simulink model "bldc_model_2018"  (R2018a)
settings: Solver=ode3  StartTime=0.0  StopTime=1  FixedStep=1e-3  MaxStep=0.0001  RelTol=1e-3  EnableMultiTasking=on
settings Model: Creator=root  LastModifiedBy=Rusty Goh
settings SolverCC: AlgebraicLoopSolver=LineSearch
settings DataIOCC: LimitDataPoints=on  SaveFormat=Array
settings OptimizationCC: LifeSpan=inf
settings DebuggingCC: SolverPrmCheckMsg=warning  SFUnexpectedBacktrackingDiag=warning  SFNoUnconditionalDefaultTransitionDiag=warning  SFExecutionAtInitializationDiag=none
settings HardwareCC: ProdBitPerPointer=32  ProdBitPerSizeT=32  ProdBitPerPtrDiffT=32  ProdLargestAtomicFloat=None  ProdIntDivRoundTo=Undefined  ProdEndianess=Unspecified  ProdWordSize=32  ProdHWDeviceType=32-bit Generic
settings ModelReferenceCC: PropagateSignalLabelsOutOfModel=off
settings CodeAppCC: StateflowObjectComments=on
settings GRTTargetCC: TargetLangStandard=C89/C90 (ANSI)  GeneratePreprocessorConditionals=Disable all
settings ConfigComp: CovMetricSettings=dw  CovHtmlReporting=on  CovSaveCumulativeToWorkspaceVar=on  CovSaveSingleToWorkspaceVar=on  CovExternalEMLEnable=off  CovSFcnEnable=off

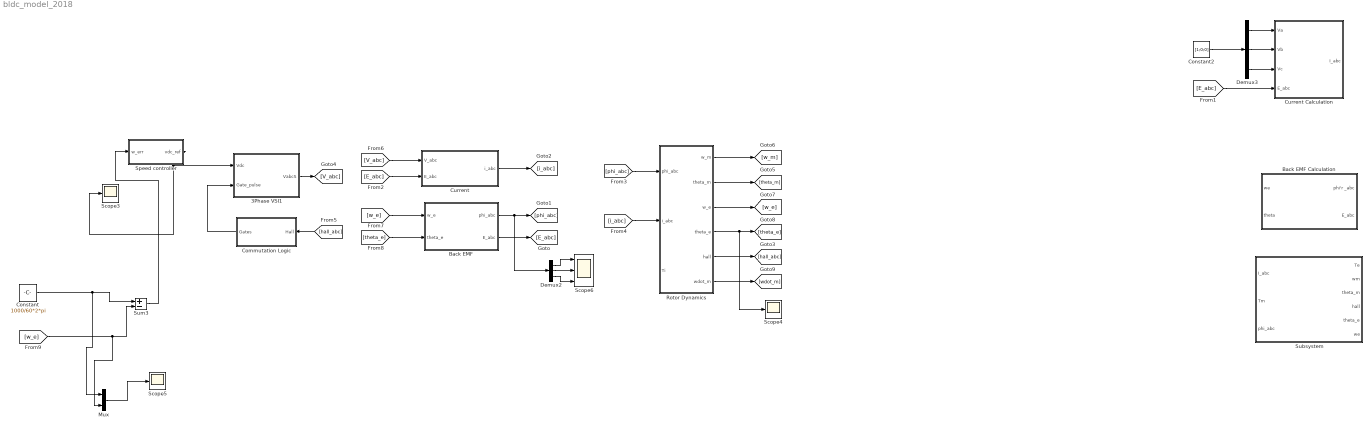
== system bldc_model_2018 ==
  3Phase VSI1 : Subsystem
  Back EMF : Subsystem
  Back EMF Calculation : Subsystem  mask{ke=0.2158/.5, trap=0.5, flux=0.2158}
  Commutation Logic : Subsystem
  Constant : Constant  Value=1000/60*2*pi
  Constant2 : Constant  Value=[1;0;0]  VectorParams1D=off
  Current : Subsystem
  Current Calculation : Subsystem  mask{Rs=1.43, Ls=9.4e-3}
      mask prompts: Rs "Resistance"; Ls "Inductance"
  Demux2 : Demux  Outputs=3
  Demux3 : Demux  Outputs=3
  Mux : Mux  Inputs=2
  Rotor Dynamics : Subsystem  mask{p=4}
      mask prompts: p "poles"
  Scope3 : Scope
  Scope4 : Scope
  Scope5 : Scope
  Scope6 : Scope  NumInputPorts=3
  Speed controller : Subsystem
  Subsystem : Subsystem  mask{p=4, J=1.5e-3, B=2e-3}
      mask prompts: p "poles"; J "Inertia"; B "Friction dynamic"
  Sum3 : Sum  Inputs=+-
  wires:
  [E_abc] -> Current Calculation/4(E_abc)
  Demux3/2 -> Current Calculation/2(Vb)
  Demux3/3 -> Current Calculation/3(Vc)
  Demux3/1 -> Current Calculation/1(Va)
  Constant2/1 -> Demux3/1
  [E_abc] -> Current/2(E_abc)
  Back EMF/2(E_abc) -> [E_abc]
  Back EMF/1(phi_abc) -> Demux2/1, [phi_abc]
  [phi_abc] -> Rotor Dynamics/1(phi_abc)
  [i_abc] -> Rotor Dynamics/2(i_abc)
  Current/1(i_abc) -> [i_abc]
  Rotor Dynamics/5(hall) -> [hall_abc]
  Commutation Logic/1(Gates) -> 3Phase VSI1/2(Gate_pulse)
  [V_abc] -> Current/1(V_abc)
  Rotor Dynamics/2(theta_m) -> [theta_m]
  Rotor Dynamics/1(w_m) -> [w_m]
  Rotor Dynamics/3(w_e) -> [w_e]
  Rotor Dynamics/4(theta_e) -> Scope4/1, [theta_e]
  [theta_e] -> Back EMF/2(theta_e)
  [w_e] -> Back EMF/1(w_e)
  3Phase VSI1/1(VabcS) -> [V_abc]
  [hall_abc] -> Commutation Logic/1("Hall ")
  Sum3/1 -> Speed controller/1(w_err)
  Speed controller/1(vdc_ref) -> Scope3/1, 3Phase VSI1/1(Vdc)
  Constant/1 -> Mux/1, Sum3/1
  Rotor Dynamics/6(wdot_m) -> [wdot_m]
  [w_e] -> Mux/2, Sum3/2
  Demux2/2 -> Scope6/2
  Demux2/1 -> Scope6/1
  Demux2/3 -> Scope6/3
  Mux/1 -> Scope5/1

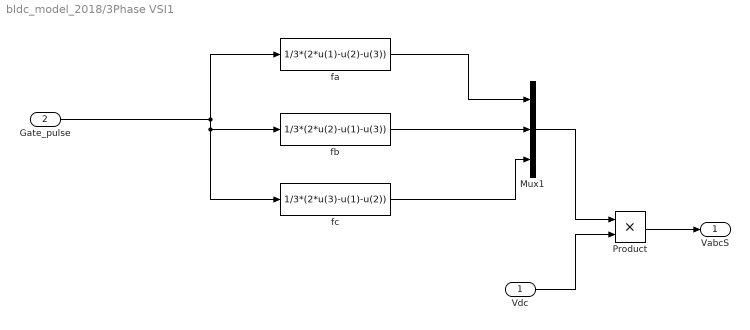
== system bldc_model_2018/3Phase VSI1 ==
  Vdc : Inport
  Gate_pulse : Inport  Port=2
  Mux1 : Mux  Inputs=3
  Product : Product
  fa : Fcn  Expr=1/3*(2*u(1)-u(2)-u(3))
  fb : Fcn  Expr=1/3*(2*u(2)-u(1)-u(3))
  fc : Fcn  Expr=1/3*(2*u(3)-u(1)-u(2))
  VabcS : Outport
  wires:
  Gate_pulse/1 -> fa/1, fb/1, fc/1
  fb/1 -> Mux1/2
  fc/1 -> Mux1/3
  fa/1 -> Mux1/1
  Mux1/1 -> Product/1
  Product/1 -> VabcS/1
  Vdc/1 -> Product/2

== system bldc_model_2018/Back EMF ==
  w_e : Inport
  theta_e : Inport  Port=2
  Back Emf : MATLABFcn  MATLABFcn=bldc_backemf  OutputDimensions=[6,1]  Output1D=off
  Demux : Demux  Outputs=[3 3]
  Mux : Mux  Inputs=[1;1]
  phi_abc : Outport
  E_abc : Outport  Port=2
  wires:
  Demux/2 -> E_abc/1
  Demux/1 -> phi_abc/1
  w_e/1 -> Mux/1
  Back Emf/1 -> Demux/1
  Mux/1 -> Back Emf/1
  theta_e/1 -> Mux/2

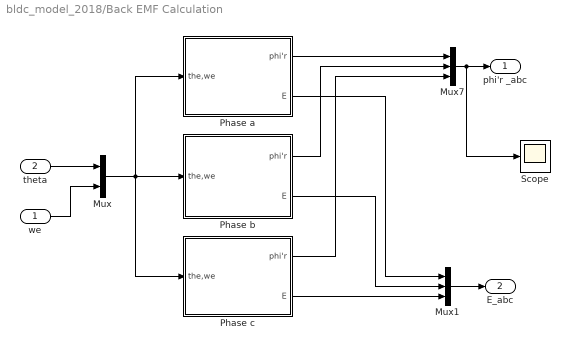
== system bldc_model_2018/Back EMF Calculation ==
  we : Inport
  theta : Inport  Port=2
  Mux : Mux  Inputs=2
  Mux1 : Mux  Inputs=3
  Mux7 : Mux  Inputs=3
  Phase a : Subsystem
  Phase b : Subsystem
  Phase c : Subsystem
  Scope : Scope
  phi'r _abc : Outport
  E_abc : Outport  Port=2
  wires:
  Mux1/1 -> E_abc/1
  Phase c/2(E) -> Mux1/3
  Phase b/2(E) -> Mux1/2
  Phase a/2(E) -> Mux1/1
  we/1 -> Mux/2
  theta/1 -> Mux/1
  Mux/1 -> Phase c/1(the,we), Phase b/1(the,we), Phase a/1(the,we)
  Phase a/1(phi'r) -> Mux7/1
  Phase b/1(phi'r) -> Mux7/2
  Phase c/1(phi'r) -> Mux7/3
  Mux7/1 -> Scope/1, phi'r _abc/1

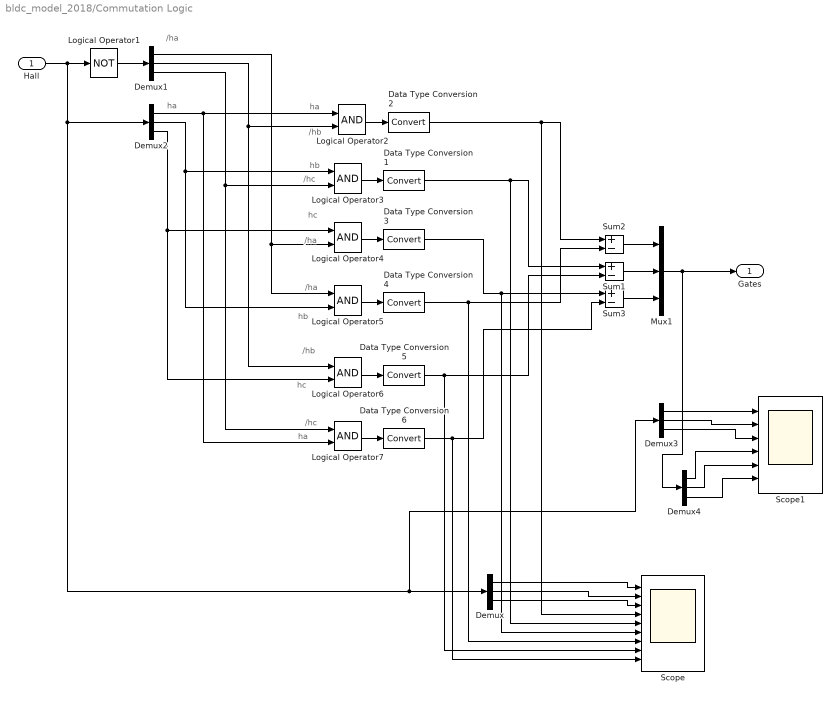
== system bldc_model_2018/Commutation Logic ==
  note: ha
  note: /hc
  note: hc
  note: /hb
  note: hb
  note: /ha
  note: /ha
  note: hc
  note: /hc
  note: hb
  note: /hb
  note: ha
  note: ha
  note: /ha
  "Hall " : Inport
  Data Type Conversion{1..6} (6 alike) : DataTypeConversion
  Demux{,1..4} (5 alike) : Demux  Outputs=3
  Logical Operator1 : Logic  Operator=NOT  AllPortsSameDT=off  OutDataTypeStr=boolean
  Logical Operator{2..7} (6 alike) : Logic  AllPortsSameDT=off  OutDataTypeStr=boolean
  Mux1 : Mux  Inputs=3
  Scope : Scope  NumInputPorts=9
  Scope1 : Scope  NumInputPorts=6
  Sum1 : Sum  Inputs=+-  OutDataTypeStr=double
  Sum2 : Sum  Inputs=+-  OutDataTypeStr=double
  Sum3 : Sum  Inputs=+-  OutDataTypeStr=double
  Gates : Outport
  wires:
  Demux2/3 -> Logical Operator6/2, Logical Operator4/1
  Sum2/1 -> Mux1/1
  Mux1/1 -> Demux4/1, Gates/1
  Logical Operator1/1 -> Demux1/1
  Logical Operator7/1 -> Data Type Conversion6/1
  Sum3/1 -> Mux1/3
  Logical Operator4/1 -> Data Type Conversion3/1
  Data Type Conversion4/1 -> Scope/7, Sum2/2
  Data Type Conversion5/1 -> Scope/8, Sum1/2
  Demux1/1 -> Logical Operator5/1, Logical Operator4/2
  Data Type Conversion3/1 -> Scope/6, Sum3/1
  Data Type Conversion6/1 -> Scope/9, Sum3/2
  Logical Operator5/1 -> Data Type Conversion4/1
  Data Type Conversion2/1 -> Scope/4, Sum2/1
  Logical Operator6/1 -> Data Type Conversion5/1
  Demux1/2 -> Logical Operator6/1, Logical Operator2/2
  Logical Operator2/1 -> Data Type Conversion2/1
  Logical Operator3/1 -> Data Type Conversion1/1
  "Hall "/1 -> Demux3/1, Demux/1, Demux2/1, Logical Operator1/1
  Data Type Conversion1/1 -> Scope/5, Sum1/1
  Sum1/1 -> Mux1/2
  Demux2/2 -> Logical Operator5/2, Logical Operator3/1
  Demux1/3 -> Logical Operator7/1, Logical Operator3/2
  Demux2/1 -> Logical Operator7/2, Logical Operator2/1
  Demux/2 -> Scope/2
  Demux/3 -> Scope/3
  Demux/1 -> Scope/1
  Demux3/1 -> Scope1/1
  Demux3/2 -> Scope1/2
  Demux3/3 -> Scope1/3
  Demux4/3 -> Scope1/6
  Demux4/2 -> Scope1/5
  Demux4/1 -> Scope1/4

== system bldc_model_2018/Current ==
  V_abc : Inport
  E_abc : Inport  Port=2
  Current : MATLABFcn  MATLABFcn=bldc_current  OutputDimensions=[3,1]  Output1D=off
  Integrator1 : Integrator  InitialCondition=[0;0;0]
  Mux1 : Mux  Inputs=[3;3;3]
  i_abc : Outport
  wires:
  Mux1/1 -> Current/1
  Current/1 -> Integrator1/1
  E_abc/1 -> Mux1/2
  Integrator1/1 -> i_abc/1, Mux1/3
  V_abc/1 -> Mux1/1

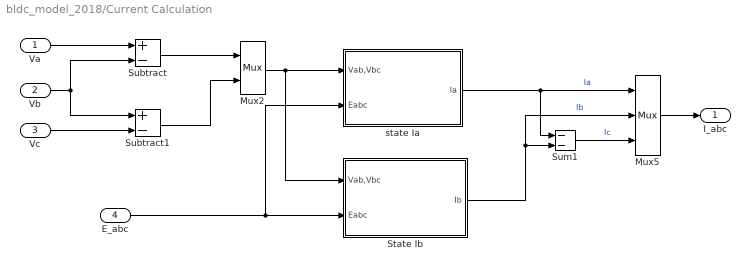
== system bldc_model_2018/Current Calculation ==
  Va : Inport
  Vb : Inport  Port=2
  Vc : Inport  Port=3
  E_abc : Inport  Port=4
  Mux2 : Mux  Inputs=2
      settings: DisplayOption=signals
  Mux5 : Mux  Inputs=3
      settings: DisplayOption=signals
  State Ib : Subsystem
  Subtract : Sum  Inputs=+-
  Subtract1 : Sum  Inputs=+-
  Sum1 : Sum  Inputs=--  SaturateOnIntegerOverflow=on
  state Ia : Subsystem
  I_abc : Outport
  wires:
  State Ib/1(Ib) -> Sum1/2, Mux5/2  "Ib"
  Subtract1/1 -> Mux2/2
  Subtract/1 -> Mux2/1
  Vc/1 -> Subtract1/2
  Vb/1 -> Subtract1/1, Subtract/2
  Va/1 -> Subtract/1
  state Ia/1(Ia) -> Mux5/1, Sum1/1  "Ia"
  Sum1/1 -> Mux5/3  "Ic"
  Mux5/1 -> I_abc/1
  Mux2/1 -> State Ib/1(Vab,Vbc), state Ia/1(Vab,Vbc)
  E_abc/1 -> state Ia/2(Eabc), State Ib/2(Eabc)

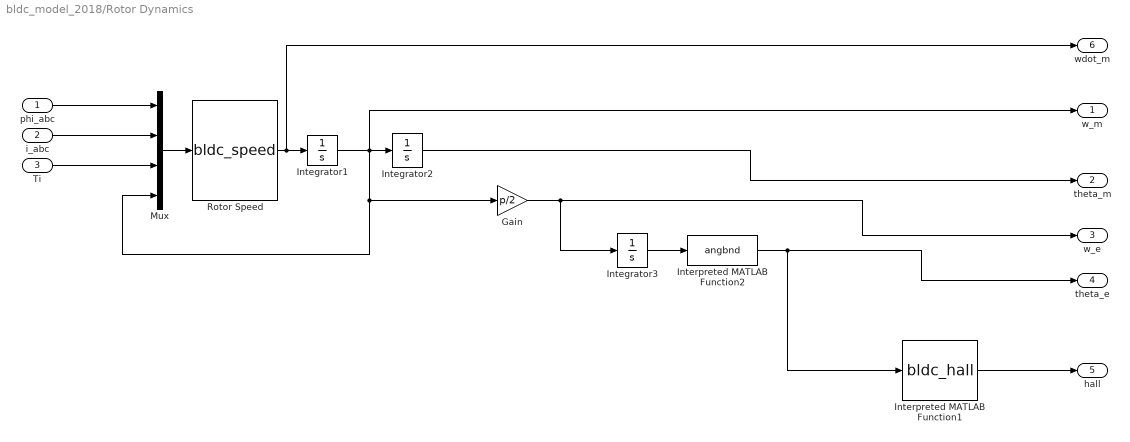
== system bldc_model_2018/Rotor Dynamics ==
  phi_abc : Inport
  i_abc : Inport  Port=2
  Ti : Inport  Port=3
  Gain : Gain  Gain=p/2
  Integrator1 : Integrator
  Integrator2 : Integrator
  Integrator3 : Integrator
  Interpreted MATLAB Function1 : MATLABFcn  MATLABFcn=bldc_hall  Output1D=off
  Interpreted MATLAB Function2 : MATLABFcn  MATLABFcn=angbnd
  Mux : Mux  Inputs=[3;3;1;1]
  Rotor Speed : MATLABFcn  MATLABFcn=bldc_speed  OutputDimensions=[1,1]  Output1D=off
  w_m : Outport
  theta_m : Outport  Port=2
  w_e : Outport  Port=3
  theta_e : Outport  Port=4
  hall : Outport  Port=5
  wdot_m : Outport  Port=6
  wires:
  Rotor Speed/1 -> wdot_m/1, Integrator1/1
  Ti/1 -> Mux/3
  i_abc/1 -> Mux/2
  Integrator1/1 -> w_m/1, Gain/1, Mux/4, Integrator2/1
  Mux/1 -> Rotor Speed/1
  Gain/1 -> Integrator3/1, w_e/1
  phi_abc/1 -> Mux/1
  Integrator2/1 -> theta_m/1
  Interpreted MATLAB Function1/1 -> hall/1
  Integrator3/1 -> Interpreted MATLAB Function2/1
  Interpreted MATLAB Function2/1 -> Interpreted MATLAB Function1/1, theta_e/1

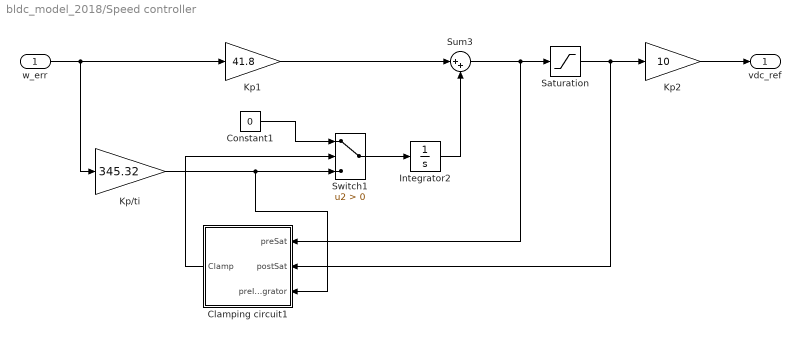
== system bldc_model_2018/Speed controller ==
  w_err : Inport
  Clamping circuit1 : Subsystem
  Constant1 : Constant  DisableCoverage=on  Value=0  OutDataTypeStr=Inherit: Inherit via back propagation  PreserveConstantTs=on
  Integrator2 : Integrator
  Kp/ti : Gain  Gain=345.32
  Kp1 : Gain  Gain=41.8
  Kp2 : Gain  Gain=10
  Saturation : Saturate  UpperLimit=15  LowerLimit=-15
  Sum3 : Sum  Inputs=|++
  Switch1 : Switch  DisableCoverage=on  Criteria=u2 > Threshold  InputSameDT=on
  vdc_ref : Outport
  wires:
  Kp1/1 -> Sum3/1
  Sum3/1 -> Saturation/1, Clamping circuit1/1(preSat)
  Saturation/1 -> Kp2/1, Clamping circuit1/2(postSat)
  w_err/1 -> Kp/ti/1, Kp1/1
  Kp2/1 -> vdc_ref/1
  Integrator2/1 -> Sum3/2
  Kp/ti/1 -> Switch1/3, Clamping circuit1/3(preIntegrator)
  Clamping circuit1/1(Clamp) -> Switch1/2
  Switch1/1 -> Integrator2/1
  Constant1/1 -> Switch1/1

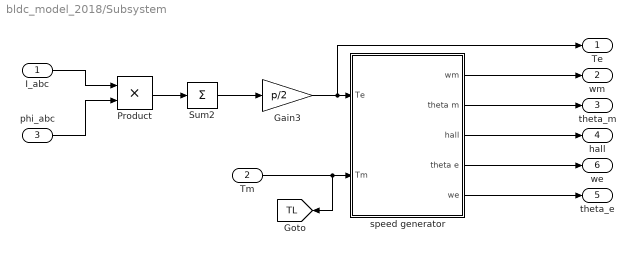
== system bldc_model_2018/Subsystem ==
  I_abc : Inport
  Tm : Inport  Port=2
  phi_abc : Inport  Port=3
  Gain3 : Gain  Gain=p/2  SaturateOnIntegerOverflow=on  OutDataTypeStr=Inherit: Same as input  ParamDataTypeStr=Inherit: Same as input
  Product : Product  SaturateOnIntegerOverflow=on  OutDataTypeStr=Inherit: Same as first input
  Sum2 : Sum  Inputs=+  SaturateOnIntegerOverflow=on
  speed generator : Subsystem
  Te : Outport
  wm : Outport  Port=2
  theta_m : Outport  Port=3
  hall : Outport  Port=4
  theta_e : Outport  Port=5
  we : Outport  Port=6
  tag scope: TL=global
  wires:
  I_abc/1 -> Product/1
  speed generator/4(theta e) -> we/1
  speed generator/3(hall) -> hall/1
  speed generator/2(theta m) -> theta_m/1
  speed generator/1(wm) -> wm/1
  Tm/1 -> [TL], speed generator/2(Tm)
  phi_abc/1 -> Product/2
  Product/1 -> Sum2/1
  Sum2/1 -> Gain3/1
  Gain3/1 -> Te/1, speed generator/1(Te)
  speed generator/5(we) -> theta_e/1

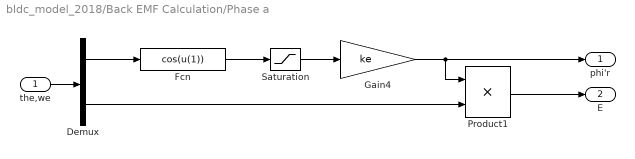
== system bldc_model_2018/Back EMF Calculation/Phase a ==
  the,we : Inport
  Demux : Demux  Outputs=2
  Fcn : Fcn  Expr=cos(u(1))
  Gain4 : Gain  Gain=ke  SaturateOnIntegerOverflow=on  OutDataTypeStr=Inherit: Same as input  ParamDataTypeStr=Inherit: Same as input
  Product1 : Product  SaturateOnIntegerOverflow=on  OutDataTypeStr=Inherit: Same as first input
  Saturation : Saturate  UpperLimit=trap  LowerLimit=-trap
  phi'r : Outport
  E : Outport  Port=2
  wires:
  Fcn/1 -> Saturation/1
  Demux/1 -> Fcn/1
  Demux/2 -> Product1/2
  the,we/1 -> Demux/1
  Product1/1 -> E/1
  Gain4/1 -> phi'r/1, Product1/1
  Saturation/1 -> Gain4/1

== system bldc_model_2018/Back EMF Calculation/Phase b ==
  note: Phi' r
  the,we : Inport
  Demux : Demux  Outputs=2
  Fcn : Fcn  Expr=cos(u(1)-2*pi/3)
  Gain4 : Gain  Gain=flux/trap  SaturateOnIntegerOverflow=on  OutDataTypeStr=Inherit: Same as input  ParamDataTypeStr=Inherit: Same as input
  Product1 : Product  SaturateOnIntegerOverflow=on  OutDataTypeStr=Inherit: Same as first input
  Saturation : Saturate  UpperLimit=trap  LowerLimit=-trap
  phi'r : Outport
  E : Outport  Port=2
  wires:
  Fcn/1 -> Saturation/1
  Saturation/1 -> Gain4/1
  Gain4/1 -> Product1/1, phi'r/1
  Product1/1 -> E/1
  the,we/1 -> Demux/1
  Demux/2 -> Product1/2
  Demux/1 -> Fcn/1

== system bldc_model_2018/Back EMF Calculation/Phase c ==
  note: Phi' r
  the,we : Inport
  Demux : Demux  Outputs=2
  Fcn : Fcn  Expr=cos(u(1)+2*pi/3)
  Gain4 : Gain  Gain=flux/trap  SaturateOnIntegerOverflow=on  OutDataTypeStr=Inherit: Same as input  ParamDataTypeStr=Inherit: Same as input
  Product1 : Product  SaturateOnIntegerOverflow=on  OutDataTypeStr=Inherit: Same as first input
  Saturation : Saturate  UpperLimit=trap  LowerLimit=-trap
  phi'r : Outport
  E : Outport  Port=2
  wires:
  Fcn/1 -> Saturation/1
  Saturation/1 -> Gain4/1
  Demux/1 -> Fcn/1
  Demux/2 -> Product1/2
  the,we/1 -> Demux/1
  Product1/1 -> E/1
  Gain4/1 -> phi'r/1, Product1/1

== system bldc_model_2018/Current Calculation/State Ib ==
  Vab,Vbc : Inport
  Eabc : Inport  Port=2
  Fcn : Fcn  Expr=-u(1)+u(2)+u(3)-2*u(4)+u(5)-3*Rs*u(6)
  Gain2 : Gain  Gain=1/(3*Ls)  SaturateOnIntegerOverflow=on  OutDataTypeStr=Inherit: Same as input  ParamDataTypeStr=Inherit: Same as input
  Mux : Mux  Inputs=3
  "s " : Integrator
  Ib : Outport
  wires:
  "s "/1 -> Ib/1, Mux/3
  Fcn/1 -> Gain2/1
  Mux/1 -> Fcn/1
  Eabc/1 -> Mux/2
  Vab,Vbc/1 -> Mux/1
  Gain2/1 -> "s "/1

== system bldc_model_2018/Current Calculation/state Ia ==
  Vab,Vbc : Inport
  Eabc : Inport  Port=2
  Gain2 : Gain  Gain=1/(3*Ls)  SaturateOnIntegerOverflow=on  OutDataTypeStr=Inherit: Same as input  ParamDataTypeStr=Inherit: Same as input
  Idot_a = 2*Vab+Vbc-2*Ea+Eb+Ec-3*Rs*ia : Fcn  Expr=2*u(1)+u(2)-2*u(3)+u(4)+u(5)-3*Rs*u(6)
  Mux : Mux  Inputs=3
  "s " : Integrator
  Ia : Outport
  wires:
  Gain2/1 -> "s "/1
  Vab,Vbc/1 -> Mux/1
  Eabc/1 -> Mux/2
  Mux/1 -> Idot_a = 2*Vab+Vbc-2*Ea+Eb+Ec-3*Rs*ia/1
  Idot_a = 2*Vab+Vbc-2*Ea+Eb+Ec-3*Rs*ia/1 -> Gain2/1
  "s "/1 -> Ia/1, Mux/3

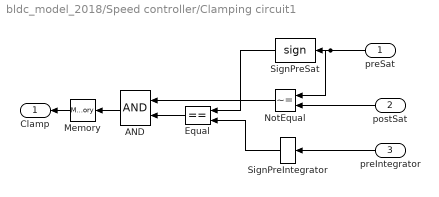
== system bldc_model_2018/Speed controller/Clamping circuit1 ==
  preSat : Inport
  postSat : Inport  Port=2
  preIntegrator : Inport  Port=3
  AND : Logic  DisableCoverage=on  OutDataTypeStr=boolean
  Equal : RelationalOperator  DisableCoverage=on  Operator===  OutDataTypeStr=boolean  RndMeth=Nearest  InputSameDT=on
  Memory : Memory
  NotEqual : RelationalOperator  DisableCoverage=on  Operator=~=  OutDataTypeStr=boolean  RndMeth=Nearest  InputSameDT=on
  SignPreIntegrator : Signum  DisableCoverage=on
  SignPreSat : Signum  DisableCoverage=on
  Clamp : Outport
  wires:
  Memory/1 -> Clamp/1
  AND/1 -> Memory/1
  Equal/1 -> AND/2
  SignPreIntegrator/1 -> Equal/2
  NotEqual/1 -> AND/1
  SignPreSat/1 -> Equal/1
  preIntegrator/1 -> SignPreIntegrator/1
  postSat/1 -> NotEqual/2
  preSat/1 -> NotEqual/1, SignPreSat/1

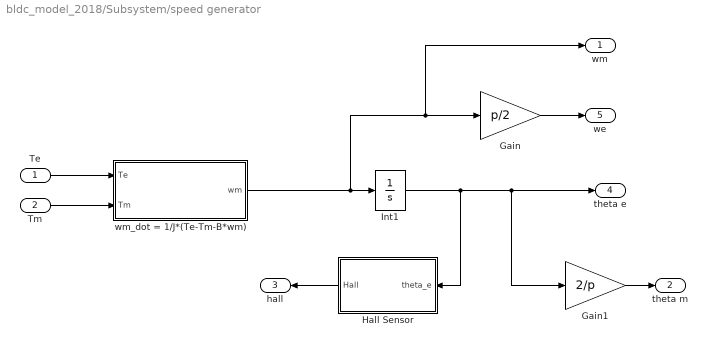
== system bldc_model_2018/Subsystem/speed generator ==
  Te : Inport
  Tm : Inport  Port=2
  Gain : Gain  Gain=p/2  SaturateOnIntegerOverflow=on  OutDataTypeStr=Inherit: Same as input  ParamDataTypeStr=Inherit: Same as input
  Gain1 : Gain  Gain=2/p  SaturateOnIntegerOverflow=on  OutDataTypeStr=Inherit: Same as input  ParamDataTypeStr=Inherit: Same as input
  Hall Sensor : Subsystem
  Int1 : Integrator
  wm_dot = 1/J*(Te-Tm-B*wm) : Subsystem
  wm : Outport
  theta m : Outport  Port=2
  hall : Outport  Port=3
  theta e : Outport  Port=4
  we : Outport  Port=5
  wires:
  Gain1/1 -> theta m/1
  Hall Sensor/1(Hall) -> hall/1
  wm_dot = 1/J*(Te-Tm-B*wm)/1("wm ") -> wm/1, Gain/1, Int1/1
  Int1/1 -> Gain1/1, theta e/1, Hall Sensor/1(theta_e)
  Te/1 -> wm_dot = 1/J*(Te-Tm-B*wm)/1(Te)
  Tm/1 -> wm_dot = 1/J*(Te-Tm-B*wm)/2(Tm)
  Gain/1 -> we/1

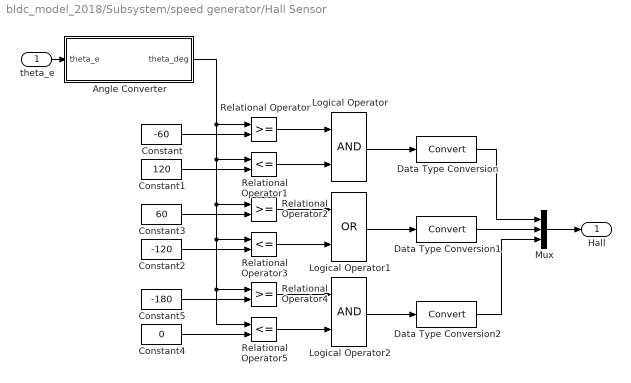
== system bldc_model_2018/Subsystem/speed generator/Hall Sensor ==
  theta_e : Inport
  Angle Converter : Subsystem
  Constant : Constant  Value=-60
  Constant1 : Constant  Value=120
  Constant2 : Constant  Value=-120
  Constant3 : Constant  Value=60
  Constant4 : Constant  Value=0
  Constant5 : Constant  Value=-180
  Data Type Conversion : DataTypeConversion
  Data Type Conversion1 : DataTypeConversion
  Data Type Conversion2 : DataTypeConversion
  Logical Operator : Logic  AllPortsSameDT=off  OutDataTypeStr=boolean
  Logical Operator1 : Logic  Operator=OR  AllPortsSameDT=off  OutDataTypeStr=boolean
  Logical Operator2 : Logic  AllPortsSameDT=off  OutDataTypeStr=boolean
  Mux : Mux  Inputs=3
  Relational Operator : RelationalOperator  OutDataTypeStr=boolean  RndMeth=Nearest
  Relational Operator1 : RelationalOperator  Operator=<=  OutDataTypeStr=boolean  RndMeth=Nearest
  Relational Operator2 : RelationalOperator  OutDataTypeStr=boolean  RndMeth=Nearest
  Relational Operator3 : RelationalOperator  Operator=<=  OutDataTypeStr=boolean  RndMeth=Nearest
  Relational Operator4 : RelationalOperator  OutDataTypeStr=boolean  RndMeth=Nearest
  Relational Operator5 : RelationalOperator  Operator=<=  OutDataTypeStr=boolean  RndMeth=Nearest
  Hall : Outport
  wires:
  Mux/1 -> Hall/1
  Data Type Conversion2/1 -> Mux/3
  Data Type Conversion1/1 -> Mux/2
  Data Type Conversion/1 -> Mux/1
  Logical Operator/1 -> Data Type Conversion/1
  Logical Operator1/1 -> Data Type Conversion1/1
  Logical Operator2/1 -> Data Type Conversion2/1
  Relational Operator5/1 -> Logical Operator2/2
  Relational Operator4/1 -> Logical Operator2/1
  Relational Operator3/1 -> Logical Operator1/2
  Relational Operator2/1 -> Logical Operator1/1
  Relational Operator1/1 -> Logical Operator/2
  Relational Operator/1 -> Logical Operator/1
  Constant4/1 -> Relational Operator5/2
  Constant5/1 -> Relational Operator4/2
  Constant2/1 -> Relational Operator3/2
  Constant3/1 -> Relational Operator2/2
  Constant1/1 -> Relational Operator1/2
  Constant/1 -> Relational Operator/2
  Angle Converter/1(theta_deg) -> Relational Operator5/1, Relational Operator4/1, Relational Operator3/1, Relational Operator2/1, Relational Operator1/1, Relational Operator/1
  theta_e/1 -> Angle Converter/1(theta_e)

== system bldc_model_2018/Subsystem/speed generator/wm_dot = 1//J*(Te-Tm-B*wm) ==
  Te : Inport
  Tm : Inport  Port=2
  Gain2 : Gain  Gain=1/J  SaturateOnIntegerOverflow=on  OutDataTypeStr=Inherit: Same as input  ParamDataTypeStr=Inherit: Same as input
  Gain4 : Gain  Gain=B  SaturateOnIntegerOverflow=on  OutDataTypeStr=Inherit: Same as input  ParamDataTypeStr=Inherit: Same as input
  Int : Integrator
  Sum : Sum  Inputs=+--  SaturateOnIntegerOverflow=on  InputSameDT=on  OutDataTypeStr=Inherit: Same as first input
  "wm " : Outport
  wires:
  Gain2/1 -> Int/1
  Te/1 -> Sum/1
  Tm/1 -> Sum/2
  Gain4/1 -> Sum/3
  Sum/1 -> Gain2/1
  Int/1 -> "wm "/1, Gain4/1

== system bldc_model_2018/Subsystem/speed generator/Hall Sensor/Angle Converter ==
  theta_e : Inport
  Trigonometric Function : Trigonometry
  Trigonometric Function1 : Trigonometry  Operator=cos
  Trigonometric Function2 : Trigonometry  Operator=atan2
  rad2deg : Gain  Gain=180/pi
  theta_deg : Outport
  wires:
  rad2deg/1 -> theta_deg/1
  theta_e/1 -> Trigonometric Function1/1, Trigonometric Function/1
  Trigonometric Function1/1 -> Trigonometric Function2/2
  Trigonometric Function/1 -> Trigonometric Function2/1
  Trigonometric Function2/1 -> rad2deg/1
